simulink model "dowd_control"  (R2020b)
settings: Solver=VariableStepAuto  StartTime=0.0  StopTime=10.0  RelTol=1e-3
values from neighbouring files (symbols this model uses):
  h = 0.01    [downright.m]
  K = lqr(A, B, q, r)    [downright.m]
undefined symbols (not defined in the file or in its folder): Humusoft, MF634
libraries: simulink x4, simulink_extras x3, sldrtlib x2
settings Model: Creator=zhehanli  LastModifiedBy=zhehanli

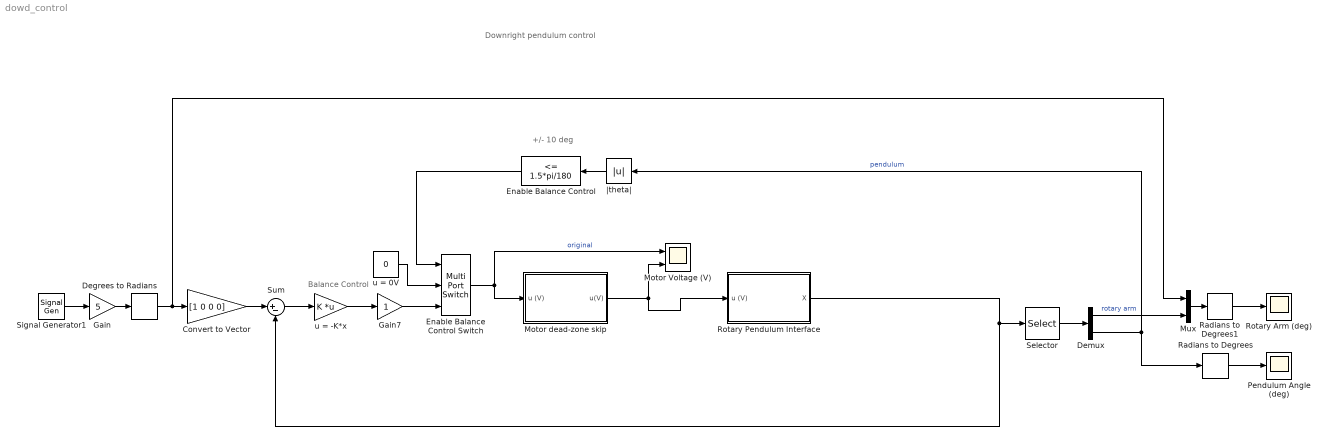
== system dowd_control ==
  note: +/- 10 deg
  note: Balance Control
  note: Downright pendulum control
  Convert to Vector : Gain  Gain=[1 0 0 0]
  Degrees to Radians : simulink_extras/Transformations/Degrees to Radians
  Demux : Demux  Outputs=2
  Enable Balance Control : simulink/Logic and Bit Operations/Compare To Constant  relop=<=  const=1.5*pi/180  OutDataTypeStr=uint8  ZeroCross=off
  Enable Balance Control Switch : MultiPortSwitch  DataPortOrder=Zero-based contiguous  Inputs=2  zeroidx=on
  Gain : Gain  Gain=5
  Gain7 : Gain
  Motor Voltage (V) : Scope  NumInputPorts=2
  Motor dead-zone skip : Subsystem
  Mux : Mux  Inputs=2
  Pendulum Angle (deg) : Scope
  Radians to Degrees : simulink_extras/Transformations/Radians to Degrees
  Radians to Degrees1 : simulink_extras/Transformations/Radians to Degrees
  Rotary Arm (deg) : Scope
  Rotary Pendulum Interface : Subsystem
  Selector : Selector  InputPortWidth=4  IndexOptions=Index vector (dialog)  Indices=[1 2]  OutputSizes=1
  Signal Generator1 : SignalGenerator  WaveForm=square  Frequency=0.1
  Sum : Sum  Inputs=|+-
  u = -K*x : Gain  Gain=K  Multiplication=Matrix(K*u)
  u = 0V : Constant  Value=0
  |theta| : Abs
  wires:
  Signal Generator1/1 -> Gain/1
  Enable Balance Control/1 -> Enable Balance Control Switch/1
  Demux/2 -> Radians to Degrees/1, |theta|/1  "pendulum"
  Motor dead-zone skip/1(u(V)) -> Rotary Pendulum Interface/1(u (V)), Motor Voltage (V)/2
  Selector/1 -> Demux/1
  Gain7/1 -> Enable Balance Control Switch/3
  Enable Balance Control Switch/1 -> Motor Voltage (V)/1, Motor dead-zone skip/1(u (V))  "original"
  Radians to Degrees/1 -> Pendulum Angle (deg)/1
  Gain/1 -> Degrees to Radians/1
  |theta|/1 -> Enable Balance Control/1
  Mux/1 -> Radians to Degrees1/1
  u = 0V/1 -> Enable Balance Control Switch/2
  Sum/1 -> u = -K*x/1
  Convert to Vector/1 -> Sum/1
  Rotary Pendulum Interface/1(X) -> Sum/2, Selector/1
  Degrees to Radians/1 -> Mux/1, Convert to Vector/1
  Radians to Degrees1/1 -> Rotary Arm (deg)/1
  u = -K*x/1 -> Gain7/1
  Demux/1 -> Mux/2  "rotary arm"

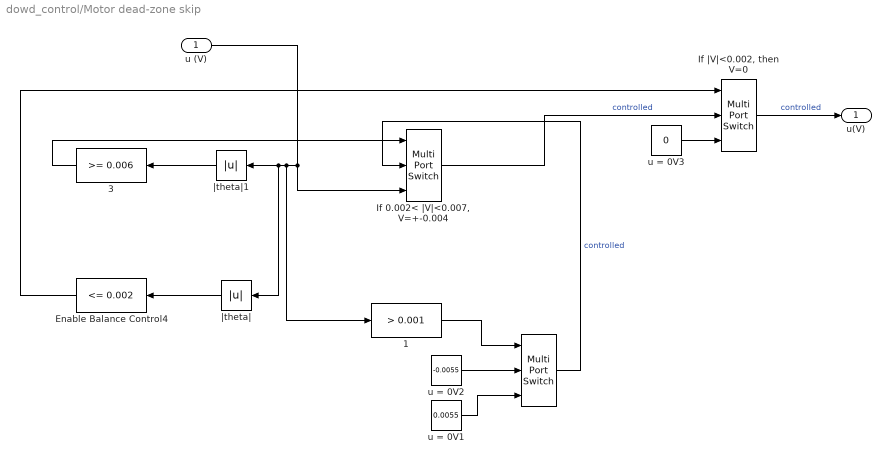
== system dowd_control/Motor dead-zone skip ==
  u (V) : Inport
  "\t" : MultiPortSwitch  DataPortOrder=Zero-based contiguous  Inputs=2  zeroidx=on
  "\tIf 0.002< |V|<0.007, V=+-0.004" : MultiPortSwitch  DataPortOrder=Zero-based contiguous  Inputs=2  zeroidx=on
  1 : simulink/Logic and Bit Operations/Compare To Constant  relop=>  const=0.001  OutDataTypeStr=uint8  ZeroCross=off
  3 : simulink/Logic and Bit Operations/Compare To Constant  relop=>=  const=0.006  OutDataTypeStr=uint8  ZeroCross=off
  Enable Balance Control4 : simulink/Logic and Bit Operations/Compare To Constant  relop=<=  const=0.002  OutDataTypeStr=uint8  ZeroCross=off
  "If |V|<0.002, then V=0" : MultiPortSwitch  DataPortOrder=Zero-based contiguous  Inputs=2  zeroidx=on
  u = 0V1 : Constant  Value=0.0055
  u = 0V2 : Constant  Value=-0.0055
  u = 0V3 : Constant  Value=0
  |theta| : Abs
  |theta|1 : Abs
  u(V) : Outport  VectorParamsAs1DForOutWhenUnconnected=off
  wires:
  "If |V|<0.002, then V=0"/1 -> u(V)/1  "controlled"
  Enable Balance Control4/1 -> "If |V|<0.002, then V=0"/1
  3/1 -> "\tIf 0.002< |V|<0.007, V=+-0.004"/1
  |theta|/1 -> Enable Balance Control4/1
  |theta|1/1 -> 3/1
  1/1 -> "\t"/1
  u = 0V1/1 -> "\t"/3
  u = 0V2/1 -> "\t"/2
  "\t"/1 -> "\tIf 0.002< |V|<0.007, V=+-0.004"/2  "controlled"
  "\tIf 0.002< |V|<0.007, V=+-0.004"/1 -> "If |V|<0.002, then V=0"/2  "controlled"
  u (V)/1 -> "\tIf 0.002< |V|<0.007, V=+-0.004"/3, |theta|/1, |theta|1/1, 1/1
  u = 0V3/1 -> "If |V|<0.002, then V=0"/3

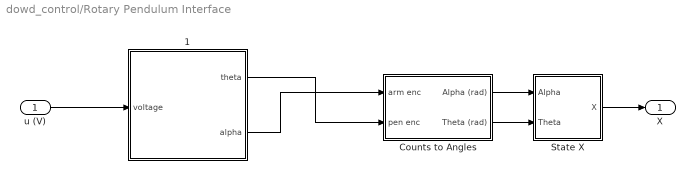
== system dowd_control/Rotary Pendulum Interface ==
  u (V) : Inport
  " 1" : Subsystem  LoadFcn=hwinit  InitFcn=hwinit  mask{h=h}
      mask prompts: h "Sampling period [s]"
      mask Display:
      | disp('Qube-Servo')
      | port_label('output',1,'theta')
      | port_label('output',2,'alpha')
      | port_label('input',1,'V')
  Counts to Angles : Subsystem
  State X : Subsystem
  X : Outport  VectorParamsAs1DForOutWhenUnconnected=off
  wires:
  u (V)/1 -> " 1"/1(voltage)
  " 1"/1(theta) -> Counts to Angles/2(pen enc)
  " 1"/2(alpha) -> Counts to Angles/1(arm enc)
  Counts to Angles/2(Theta (rad)) -> State X/2(Theta)
  Counts to Angles/1(Alpha (rad)) -> State X/1(Alpha)
  State X/1(X) -> X/1

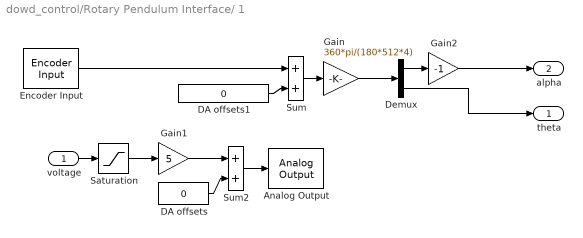
== system dowd_control/Rotary Pendulum Interface/ 1 ==
  voltage : Inport
  Analog Output : sldrtlib/Analog Output  SampleTime=h  MaxMissedTicks=100  ShowMissedTicks=off  YieldWhenWaiting=off  DrvName=Humusoft/MF634  DrvAddress=4294967295  DrvOptions=0  Channels=[1]  RangeMode=2  VoltRange=1  InitialValue=0  FinalValue=0
      settings: AttributesFormatString=Humusoft\nMF634 [auto]
  DA offsets : Constant  Value=0
  DA offsets1 : Constant  Value=0  SampleTime=h
  Demux : Demux  Outputs=2
  Encoder Input : sldrtlib/Encoder Input  SampleTime=h  MaxMissedTicks=100  ShowMissedTicks=off  YieldWhenWaiting=off  DrvName=Humusoft/MF634  DrvAddress=4294967295  DrvOptions=0  Channels=[1,2]  QuadMode=3  IndexPulse=1  InputFilter=Inf  DataType=1
      settings: AttributesFormatString=Humusoft\nMF634 [auto]
  Gain : Gain  Gain=360*pi/(180*512*4)  SaturateOnIntegerOverflow=on  OutDataTypeStr=Inherit: Same as input  ParamDataTypeStr=Inherit: Same as input
  Gain1 : Gain  Gain=5  SaturateOnIntegerOverflow=on  OutDataTypeStr=Inherit: Same as input  ParamDataTypeStr=Inherit: Same as input
  Gain2 : Gain  Gain=-1  SaturateOnIntegerOverflow=on  OutDataTypeStr=Inherit: Same as input  ParamDataTypeStr=Inherit: Same as input
  Saturation : Saturate  UpperLimit=1  LowerLimit=-1
  Sum : Sum  InputSameDT=on  SaturateOnIntegerOverflow=on  OutDataTypeStr=Inherit: Same as first input
  Sum2 : Sum  InputSameDT=on  SaturateOnIntegerOverflow=on  OutDataTypeStr=Inherit: Same as first input
  theta : Outport  Tag=Cable length
  alpha : Outport  Tag=Cable length  Port=2
  wires:
  Sum/1 -> Gain/1
  DA offsets1/1 -> Sum/2
  Gain1/1 -> Sum2/1
  Sum2/1 -> Analog Output/1
  DA offsets/1 -> Sum2/2
  voltage/1 -> Saturation/1
  Encoder Input/1 -> Sum/1
  Saturation/1 -> Gain1/1
  Demux/1 -> Gain2/1
  Gain/1 -> Demux/1
  Gain2/1 -> alpha/1
  Demux/2 -> theta/1

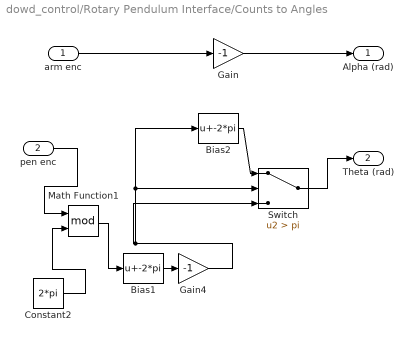
== system dowd_control/Rotary Pendulum Interface/Counts to Angles ==
  arm enc : Inport
  pen enc : Inport  Port=2
  Bias1 : Bias  Bias=-2*pi
  Bias2 : Bias  Bias=-2*pi
  Constant2 : Constant  Value=2*pi
  Gain : Gain  Gain=-1
  Gain4 : Gain  Gain=-1
  Math Function1 : Math  Operator=mod  SignedPower=on  SaturateOnIntegerOverflow=on
  Switch : Switch  Criteria=u2 > Threshold  Threshold=pi
  Alpha (rad) : Outport  VectorParamsAs1DForOutWhenUnconnected=off
  Theta (rad) : Outport  Port=2  VectorParamsAs1DForOutWhenUnconnected=off
  wires:
  arm enc/1 -> Gain/1
  Gain4/1 -> Switch/3, Switch/2, Bias2/1
  Bias2/1 -> Switch/1
  Math Function1/1 -> Bias1/1
  pen enc/1 -> Math Function1/1
  Constant2/1 -> Math Function1/2
  Bias1/1 -> Gain4/1
  Gain/1 -> Alpha (rad)/1
  Switch/1 -> Theta (rad)/1

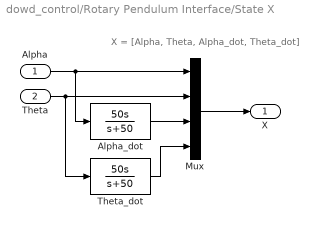
== system dowd_control/Rotary Pendulum Interface/State X ==
  note: X = [Alpha, Theta, Alpha_dot, Theta_dot]
  Alpha : Inport
  Theta : Inport  Port=2
  Alpha_dot : TransferFcn  Numerator=[50 0]  Denominator=[1 50]
  Mux : Mux
  Theta_dot : TransferFcn  Numerator=[50 0]  Denominator=[1 50]
  X : Outport  VectorParamsAs1DForOutWhenUnconnected=off
  wires:
  Alpha_dot/1 -> Mux/3
  Theta_dot/1 -> Mux/4
  Theta/1 -> Mux/2, Theta_dot/1
  Mux/1 -> X/1
  Alpha/1 -> Mux/1, Alpha_dot/1
